simulink model "Modell_V4"  (R2015b)
settings: Solver=ode45  StartTime=0.0  StopTime=0.5  RelTol=1e-3
values from neighbouring files (symbols this model uses):
  AP = modelPars(ii).AP    [Hilfsskript_sFunction.m]    (also in hilf_mir.m = [pi/3 0 0 0]; simGUI.m = [0 0 0 0])
  K = berechneLQR(A,B,Q,R)    [Hilfsskript_sFunction.m]    (also in simGUI.m = str2num(get(h.reglerK,'String')))
  M_AP = double(M_AP)    [linearisierung.m]    (also in simGUI.m = str2num(get(h.M_AP,'String')))
  stPendel = ladePendel    [Hilfsskript_sFunction.m]    (also in hilf_mir.m = ladePendel(); simGUI.m = ladePendel())
  x0 = modelPars(ii).x0    [Hilfsskript_sFunction.m]    (also in hilf_mir.m = [-pi/3 0 0 0])
undefined symbols (not defined in the file or in its folder): stObs
settings Model: Creator=asacakli  LastModifiedBy=ajentsch

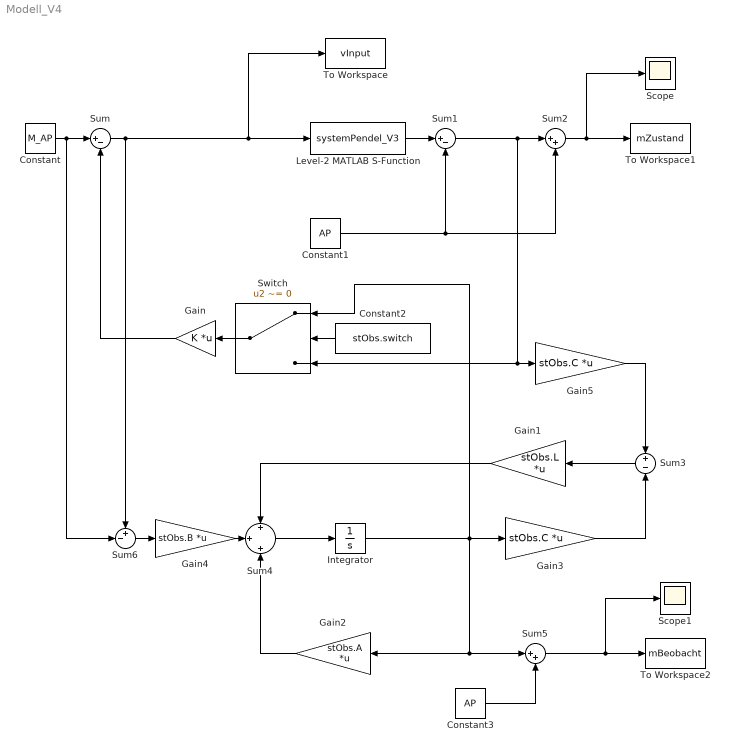
== system Modell_V4 ==
  Constant : Constant  Value=M_AP
  Constant1 : Constant  Value=AP
  Constant2 : Constant  Value=stObs.switch
  Constant3 : Constant  Value=AP
  Gain : Gain  Gain=K  Multiplication=Matrix(K*u)
  Gain1 : Gain  Gain=stObs.L  Multiplication=Matrix(K*u)
  Gain2 : Gain  Gain=stObs.A  Multiplication=Matrix(K*u)
  Gain3 : Gain  Gain=stObs.C  Multiplication=Matrix(K*u)
  Gain4 : Gain  Gain=stObs.B  Multiplication=Matrix(K*u)
  Gain5 : Gain  Gain=stObs.C  Multiplication=Matrix(K*u)
  Integrator : Integrator  InitialCondition=stObs.x0'-AP'
  Level-2 MATLAB S-Function : M-S-Function  FunctionName=systemPendel_V3  Parameters=stPendel,x0
  Scope : Scope
  Scope1 : Scope
  Sum : Sum  Inputs=|+-
  Sum1 : Sum  Inputs=|+-
  Sum2 : Sum  Inputs=|++
  Sum3 : Sum  Inputs=+|-
  Sum4 : Sum  Inputs=+|+|+
  Sum5 : Sum  Inputs=|++
  Sum6 : Sum  Inputs=+-|
  Switch : Switch  Criteria=u2 ~= 0
  To Workspace : ToWorkspace  VariableName=vInput  SaveFormat=Timeseries  SampleTime=-1
  To Workspace1 : ToWorkspace  VariableName=mZustand  SaveFormat=Timeseries  SampleTime=-1
  To Workspace2 : ToWorkspace  VariableName=mBeobacht  SaveFormat=Timeseries  SampleTime=-1
  wires:
  Constant/1 -> Sum6/2, Sum/1
  Gain/1 -> Sum/2
  Sum/1 -> Sum6/1, To Workspace/1, Level-2 MATLAB S-Function/1
  Sum1/1 -> Sum2/1, Switch/3, Gain5/1
  Constant1/1 -> Sum2/2, Sum1/2
  Level-2 MATLAB S-Function/1 -> Sum1/1
  Sum2/1 -> Scope/1, To Workspace1/1
  Switch/1 -> Gain/1
  Constant2/1 -> Switch/2
  Sum3/1 -> Gain1/1
  Sum4/1 -> Integrator/1
  Gain1/1 -> Sum4/1
  Gain2/1 -> Sum4/3
  Integrator/1 -> Sum5/1, Gain2/1, Gain3/1, Switch/1
  Gain3/1 -> Sum3/2
  Gain4/1 -> Sum4/2
  Sum6/1 -> Gain4/1
  Gain5/1 -> Sum3/1
  Sum5/1 -> Scope1/1, To Workspace2/1
  Constant3/1 -> Sum5/2
